simulink model "distributed_six"  (R2018a)
settings: Solver=VariableStepAuto  StartTime=0.0  StopTime=3000  FixedStep=0.0125  RelTol=1e-3  EnableMultiTasking=on
PreLoadFcn:
  | t_sampling = 0.1;
undefined symbols (not defined in the file or in its folder): DiscIntNeverNeededParam
settings Model: Creator=Kevin_ME813  LastModifiedBy=Kevin_ME813
settings SolverCC: ConcurrentTasks=on
settings DataIOCC: SaveFormat=Array
settings OptimizationCC: EnhancedBackFolding=on  PassReuseOutputArgsAs=Individual arguments  MaxStackSize=64  OptimizeBlockOrder=speed  DifferentSizesBufferReuse=on  OptimizationCustomize=off
settings DebuggingCC: ParameterTunabilityLossMsg=error
settings HardwareCC: ProdBitPerLong=64  ProdHWDeviceType=Intel->x86-64 (Linux 64)
settings SFSimCC: MATLABDynamicMemAlloc=off
settings RTWCC: SystemTargetFile=ert.tlc  HardwareBoard=Robot Operating System (ROS)  TLCOptions="-aInlineSetEventsForThisBaseRateFcn=TLC_FALSE -aSuppressMultiTaskScheduler=TLC_FALSE  -aRateBasedStepFcn=0"  TemplateMakefile=ert_default_tmf  GenerateReport=on  Toolchain=Catkin  IncludeHyperlinkInReport=on  LaunchReport=on  TargetLang=C++  GenerateTraceInfo=on  GenerateTraceReport=on  GenerateTraceReportSl=on  GenerateTraceReportSf=on  GenerateTraceReportEml=on
settings CodeAppCC: ForceParamTrailComments=on  IgnoreCustomStorageClasses=off  OperatorAnnotations=on  SimulinkDataObjDesc=on  SFDataObjDesc=on  InsertBlockDesc=on

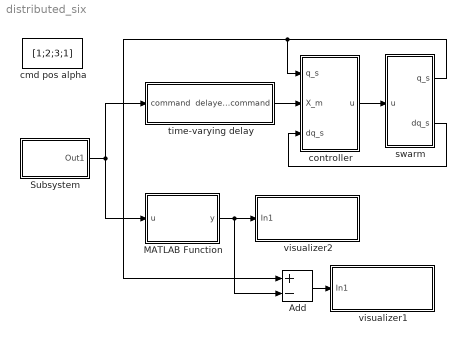
== system distributed_six ==
  Add : Sum  Inputs=+-
  MATLAB Function : MATLAB Function  TreatAsAtomicUnit=on
  Subsystem : Subsystem
  cmd pos alpha : Constant  Value=[1;2;3;1]  SampleTime=0.01
  controller : Subsystem
  swarm : Subsystem
  time-varying delay : Subsystem
  visualizer1 : Subsystem
  visualizer2 : Subsystem
  wires:
  swarm/1(q_s) -> Add/1, controller/1(q_s)
  swarm/2(dq_s) -> controller/3(dq_s)
  controller/1(u) -> swarm/1(u)
  time-varying delay/1(delayed command) -> controller/2(X_m)
  MATLAB Function/1(y) -> Add/2, visualizer2/1(In1)
  Add/1 -> visualizer1/1(In1)
  Subsystem/1(Out1) -> time-varying delay/1(command), MATLAB Function/1(u)

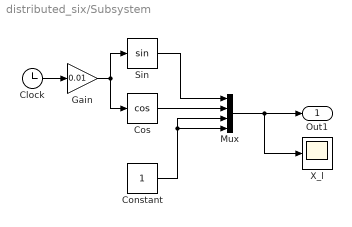
== system distributed_six/Subsystem ==
  Clock : Clock
  Constant : Constant  SampleTime=0.01
  Cos : Trigonometry  Operator=cos
  Gain : Gain  Gain=0.01
  Mux : Mux
  Sin : Trigonometry
  X_l : Scope
  Out1 : Outport
  wires:
  Mux/1 -> X_l/1, Out1/1
  Constant/1 -> Mux/3, Mux/4
  Cos/1 -> Mux/2
  Clock/1 -> Gain/1
  Sin/1 -> Mux/1
  Gain/1 -> Cos/1, Sin/1

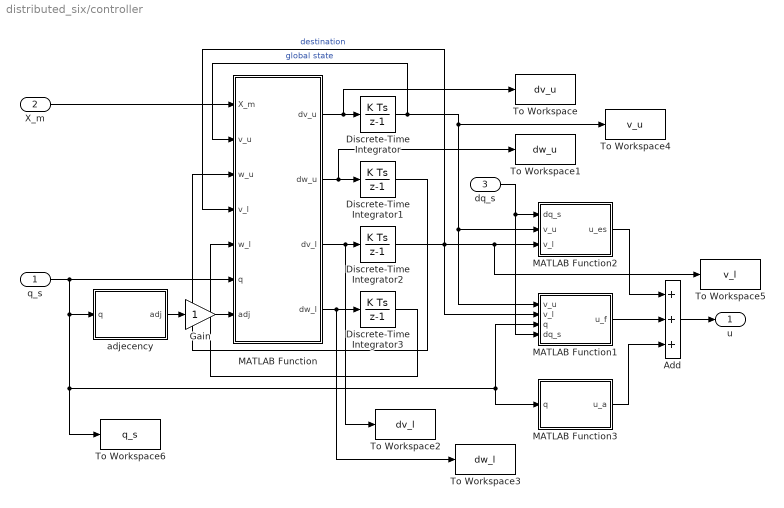
== system distributed_six/controller ==
  q_s : Inport
  X_m : Inport  Port=2
  dq_s : Inport  Port=3
  Add : Sum  Inputs=+++
  Discrete-Time Integrator{,1..3} (4 alike) : DiscreteIntegrator  SampleTime=-1  ICPrevOutput=DiscIntNeverNeededParam  ICPrevScaledInput=DiscIntNeverNeededParam
  Gain : Gain
  MATLAB Function : MATLAB Function  TreatAsAtomicUnit=on
  MATLAB Function1 : MATLAB Function  TreatAsAtomicUnit=on
  MATLAB Function2 : MATLAB Function  TreatAsAtomicUnit=on
  MATLAB Function3 : MATLAB Function  TreatAsAtomicUnit=on
  To Workspace : ToWorkspace  VariableName=dv_u  SampleTime=-1
  To Workspace1 : ToWorkspace  VariableName=dw_u  SampleTime=-1
  To Workspace2 : ToWorkspace  VariableName=dv_l  SampleTime=-1
  To Workspace3 : ToWorkspace  VariableName=dw_l  SampleTime=-1
  To Workspace4 : ToWorkspace  VariableName=v_u  SampleTime=-1
  To Workspace5 : ToWorkspace  VariableName=v_l  SampleTime=-1
  To Workspace6 : ToWorkspace  VariableName=q_s  SampleTime=-1
  adjecency : MATLAB Function  TreatAsAtomicUnit=on
  u : Outport
  wires:
  Discrete-Time Integrator1/1 -> MATLAB Function/3(w_u)
  q_s/1 -> To Workspace6/1, MATLAB Function3/1(q), MATLAB Function1/3(q), adjecency/1(q), MATLAB Function/6(q)
  Discrete-Time Integrator3/1 -> MATLAB Function/5(w_l)
  Discrete-Time Integrator2/1 -> To Workspace5/1, MATLAB Function2/3(v_l), MATLAB Function1/2(v_l), MATLAB Function/4(v_l)  "destination"
  MATLAB Function/3(dv_l) -> Discrete-Time Integrator2/1, To Workspace2/1
  MATLAB Function/4(dw_l) -> Discrete-Time Integrator3/1, To Workspace3/1
  Add/1 -> u/1
  MATLAB Function/2(dw_u) -> Discrete-Time Integrator1/1, To Workspace1/1
  Discrete-Time Integrator/1 -> To Workspace4/1, MATLAB Function1/1(v_u), MATLAB Function2/2(v_u), MATLAB Function/2(v_u)  "global state"
  MATLAB Function/1(dv_u) -> Discrete-Time Integrator/1, To Workspace/1
  MATLAB Function2/1(u_es) -> Add/1
  MATLAB Function3/1(u_a) -> Add/3
  dq_s/1 -> MATLAB Function1/4(dq_s), MATLAB Function2/1(dq_s)
  X_m/1 -> MATLAB Function/1(X_m)
  adjecency/1(adj) -> Gain/1
  Gain/1 -> MATLAB Function/7(adj)
  MATLAB Function1/1(u_f) -> Add/2

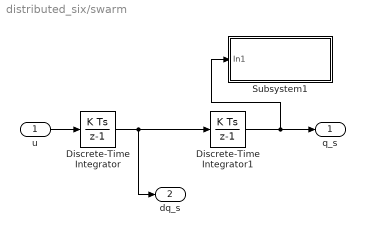
== system distributed_six/swarm ==
  u : Inport
  Discrete-Time Integrator : DiscreteIntegrator  InitialCondition=zeros(18,1)  SampleTime=-1  ICPrevOutput=DiscIntNeverNeededParam  ICPrevScaledInput=DiscIntNeverNeededParam
  Discrete-Time Integrator1 : DiscreteIntegrator  InitialCondition=[1 0 0 0.7 0.7 0 -0.7 0.7 0 -1 0 0 -0.7 -0.7 0 0.7 -0.7 0].'  SampleTime=-1  ICPrevOutput=DiscIntNeverNeededParam  ICPrevScaledInput=DiscIntNeverNeededParam
  Subsystem1 : Subsystem
  q_s : Outport
  dq_s : Outport  Port=2
  wires:
  u/1 -> Discrete-Time Integrator/1
  Discrete-Time Integrator/1 -> Discrete-Time Integrator1/1, dq_s/1
  Discrete-Time Integrator1/1 -> Subsystem1/1(In1), q_s/1

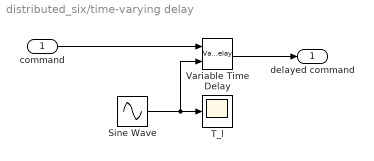
== system distributed_six/time-varying delay ==
  command : Inport
  Sine Wave : Sin  Amplitude=0.5  Bias=0.5  SampleTime=0
  T_l : Scope
  Variable Time Delay : VariableTransportDelay  MaximumDelay=5
  delayed command : Outport
  wires:
  Sine Wave/1 -> Variable Time Delay/2, T_l/1
  Variable Time Delay/1 -> delayed command/1
  command/1 -> Variable Time Delay/1

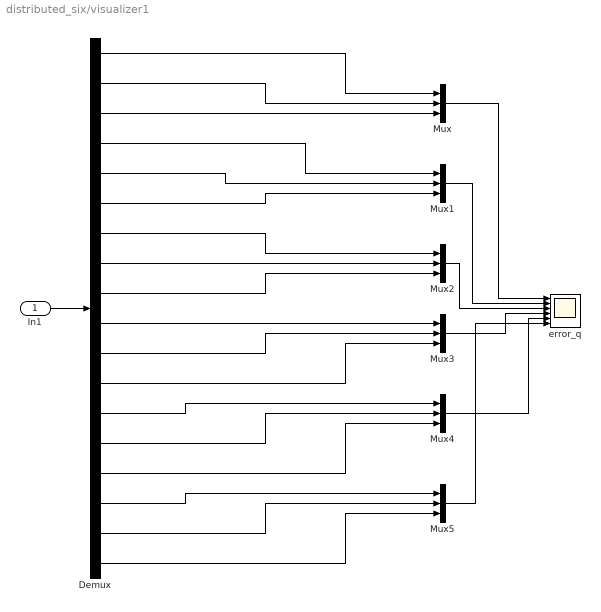
== system distributed_six/visualizer1 ==
  In1 : Inport
  Demux : Demux  Outputs=18
  Mux{,1..5} (6 alike) : Mux  Inputs=3
  error_q : Scope  NumInputPorts=6
  wires:
  Mux5/1 -> error_q/6
  Mux4/1 -> error_q/5
  Mux3/1 -> error_q/4
  Mux2/1 -> error_q/3
  Mux1/1 -> error_q/2
  Mux/1 -> error_q/1
  Demux/18 -> Mux5/3
  Demux/17 -> Mux5/2
  Demux/16 -> Mux5/1
  Demux/15 -> Mux4/3
  Demux/14 -> Mux4/2
  Demux/13 -> Mux4/1
  Demux/12 -> Mux3/3
  Demux/11 -> Mux3/2
  Demux/10 -> Mux3/1
  Demux/9 -> Mux2/3
  Demux/7 -> Mux2/1
  Demux/8 -> Mux2/2
  Demux/4 -> Mux1/1
  Demux/6 -> Mux1/3
  Demux/5 -> Mux1/2
  Demux/1 -> Mux/1
  Demux/2 -> Mux/2
  Demux/3 -> Mux/3
  In1/1 -> Demux/1

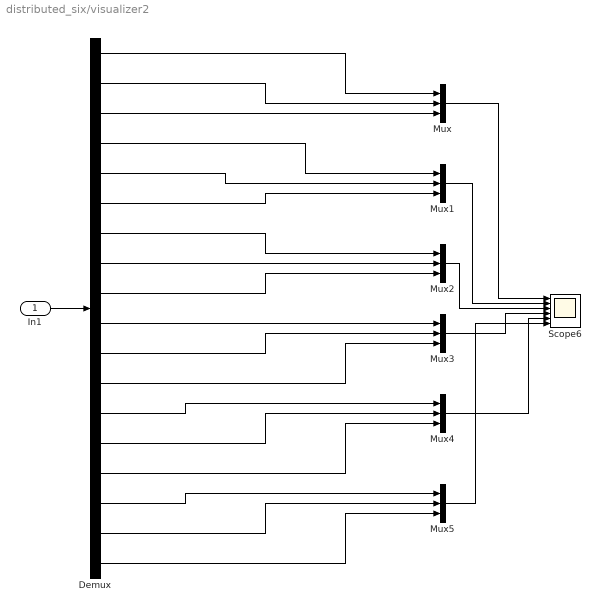
== system distributed_six/visualizer2 ==
  In1 : Inport
  Demux : Demux  Outputs=18
  Mux{,1..5} (6 alike) : Mux  Inputs=3
  Scope6 : Scope  NumInputPorts=6
  wires:
  In1/1 -> Demux/1
  Demux/3 -> Mux/3
  Demux/2 -> Mux/2
  Demux/1 -> Mux/1
  Demux/5 -> Mux1/2
  Demux/6 -> Mux1/3
  Demux/4 -> Mux1/1
  Demux/8 -> Mux2/2
  Demux/7 -> Mux2/1
  Demux/9 -> Mux2/3
  Demux/10 -> Mux3/1
  Demux/11 -> Mux3/2
  Demux/12 -> Mux3/3
  Demux/13 -> Mux4/1
  Demux/14 -> Mux4/2
  Demux/15 -> Mux4/3
  Demux/16 -> Mux5/1
  Demux/17 -> Mux5/2
  Demux/18 -> Mux5/3
  Mux/1 -> Scope6/1
  Mux1/1 -> Scope6/2
  Mux2/1 -> Scope6/3
  Mux3/1 -> Scope6/4
  Mux4/1 -> Scope6/5
  Mux5/1 -> Scope6/6

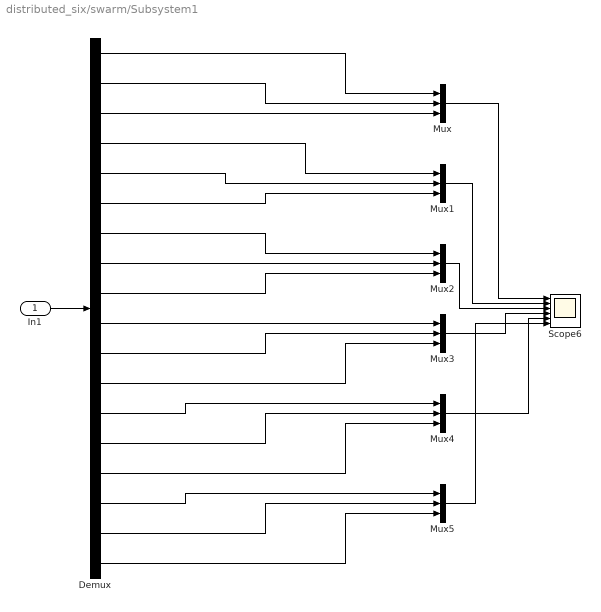
== system distributed_six/swarm/Subsystem1 ==
  In1 : Inport
  Demux : Demux  Outputs=18
  Mux{,1..5} (6 alike) : Mux  Inputs=3
  Scope6 : Scope  NumInputPorts=6
  wires:
  In1/1 -> Demux/1
  Demux/3 -> Mux/3
  Demux/2 -> Mux/2
  Demux/1 -> Mux/1
  Demux/5 -> Mux1/2
  Demux/6 -> Mux1/3
  Demux/4 -> Mux1/1
  Demux/8 -> Mux2/2
  Demux/7 -> Mux2/1
  Demux/9 -> Mux2/3
  Demux/10 -> Mux3/1
  Demux/11 -> Mux3/2
  Demux/12 -> Mux3/3
  Demux/13 -> Mux4/1
  Demux/14 -> Mux4/2
  Demux/15 -> Mux4/3
  Demux/16 -> Mux5/1
  Demux/17 -> Mux5/2
  Demux/18 -> Mux5/3
  Mux/1 -> Scope6/1
  Mux1/1 -> Scope6/2
  Mux2/1 -> Scope6/3
  Mux3/1 -> Scope6/4
  Mux4/1 -> Scope6/5
  Mux5/1 -> Scope6/6

== matlab function distributed_six/controller/adjecency ==
  data: q input; adj output
function adj = adjecency(q)
SlaveRobotNum = 6;
SlaveRobotDOF = 3;
DistanceLimit = 10;

reachable = zeros(SlaveRobotNum, SlaveRobotNum);
position = zeros(SlaveRobotNum, SlaveRobotDOF);

for num = 1 : SlaveRobotNum
    for axis = 1 : SlaveRobotDOF
        position(num, axis) = q( (num-1)*SlaveRobotDOF + axis);    
    end
end

for i = 1 : SlaveRobotNum
    for j = 1 : SlaveRobotNum
        
        if i == j
            reachable(i,j) = 0;
        elseif norm(position(i,:) - position(j,:)) <= DistanceLimit
            reachable(i,j) = 1;
        else
            reachable(i,j) = 0;
        end
    
    end
end

adj = reachable;

== matlab function distributed_six/controller/MATLAB Function ==
  data: X_m input; v_u input; dv_u output; dw_u output; w_u input; v_l input; w_l input; q input; adj input; dv_l output; dw_l output
function [dv_u,dw_u, dv_l, dw_l] = Estimator(X_m, v_u, w_u, v_l, w_l, q, adj)
SlaveRobotNum = 6;
SlaveRobotDOF = 3;
gamma = 1;
rho = 1;
k_p = 25;
k_i = 10;

dv_u = zeros(length(q),1);
dw_u = zeros(length(q),1);
dv_l = zeros(length(q)+SlaveRobotNum,1);
dw_l = zeros(length(q)+SlaveRobotNum,1);
delta = zeros(SlaveRobotNum,1);
delta(1) = 1;

for i = 1 : SlaveRobotNum   %robot number
    %index
    i1 = (i-1) * SlaveRobotDOF + 1;
    i1e = i1 + SlaveRobotDOF - 1;
    i3 = (i-1) * (SlaveRobotDOF+1) + 1;
    i3e = i3 + SlaveRobotDOF;
    
    dv_u(i1:i1e) = gamma*k_p*(q(i1:i1e) - v_u(i1:i1e));
%     dv_l(i3:i3e) = -delta(i)*k_p*(v_l(i3:i3e)-rho*X_m) + delta(i)*k_i*w_l(i3:i3e);
    dv_l(i3:i3e) = -delta(i)*k_p*(v_l(i3:i3e)-rho*X_m);
%     dw_l(i3:i3e) = -delta(i)*k_i*(v_l(i3:i3e)-rho*X_m);
    dw_l(i3:i3e) = -k_i*w_l(i3:i3e);
    
    
    for j = 1 : SlaveRobotNum   %sigma, others
        i2 = (j-1) * SlaveRobotDOF + 1;
        i2e = i2 + SlaveRobotDOF - 1;
        i4 = (j-1) * (SlaveRobotDOF+1) + 1;
        i4e = i4 + SlaveRobotDOF;
    
        if adj(i, j) ~= 0
            %3.7
            dv_u(i1:i1e) = dv_u(i1:i1e) ...
                - adj(i,j)*k_p*(v_u(i1:i1e)-v_u(i2:i2e)) ...
                + adj(i,j)*k_i*(w_u(i1:i1e)-w_u(i2:i2e));
            %3.8
            dw_u(i1:i1e) = dw_u(i1:i1e) - adj(i,j)*k_i*(v_u(i1:i1e)-v_u(i2:i2e));
            %3.9
            dv_l(i3:i3e) = dv_l(i3:i3e) ...
                - adj(i,j)*k_p*(v_l(i3:i3e)-v_l(i4:i4e)) ...
                + adj(i,j)*k_i*(w_l(i3:i3e)-w_l(i4:i4e));
            %3.10
            dw_l(i3:i3e) = dw_l(i3:i3e) - adj(i,j)*k_i*(v_l(i3:i3e)-v_l(i4:i4e));
            
        end
    end
end

== matlab function distributed_six/controller/MATLAB Function2 ==
  data: dq_s input; u_es output; v_u input; v_l input
function u_es = fcn(dq_s, v_u, v_l)
SlaveRobotNum = 6;
SlaveRobotDOF = 3;
b = ones(SlaveRobotNum, 1);
u_es = zeros(length(dq_s), 1);
Gamma = 1;
Lambda = 1;

for i = 1:SlaveRobotNum
%     index, 'e' for end
    i1 = (i-1) * SlaveRobotDOF + 1;
    i1e = i1 + SlaveRobotDOF - 1; 
    i2 = (i-1) * (SlaveRobotDOF+1) + 1;
    i2e = i2 + SlaveRobotDOF - 1;   %leading G terms
    
    u_es(i1:i1e) = -b(i)*dq_s(i1:i1e) ...
        - eye(SlaveRobotDOF)*Gamma*(v_u(i1:i1e)-v_l(i2:i2e)) ...   %eye to be modified
        - Lambda * eye(SlaveRobotDOF) * dq_s(i1:i1e);
end

== matlab function distributed_six/controller/MATLAB Function1 ==
  data: v_u input; u_f output; v_l input; q input; dq_s input
function u_f = fcn(v_u, v_l, q, dq_s)
SlaveRobotNum = 6;
SlaveRobotDOF = 3;

q_d = zeros(length(q),1);
d_f = zeros(length(q),1);
d_f(1) = 1;
u_f = zeros(length(q),1);
k_f = 1;
k_fd = 0;

for i = 1 : SlaveRobotNum   %robot number
    %index
    i1 = (i-1) * SlaveRobotDOF + 1;
    i1e = i1 + SlaveRobotDOF - 1;
    i3 = (i-1) * (SlaveRobotDOF+1) + 1;
    i3e = i3 + SlaveRobotDOF;
          
    
    q_d(i1:i1e) = v_l(i3e)*d_f(i1:i1e) + v_u(i1:i1e);
    u_f(i1:i1e) = -k_f*( q(i1:i1e)-q_d(i1:i1e) )- k_fd*dq_s(i1:i1e);
    
    if i ~= SlaveRobotNum
        d_f(i1+SlaveRobotDOF:i1e+SlaveRobotDOF) ...
            = rotz(360/SlaveRobotNum)*d_f(i1:i1e);
    end
end

== matlab function distributed_six/controller/MATLAB Function3 ==
  data: q input; u_a output
function u_a = fcn(q)

u_a = 0;

== matlab function distributed_six/MATLAB Function ==
  data: u input; y output
function y = fcn(u)

y1 = u(1:3) + u(4)*[1;0;0];
y2 = u(1:3) + u(4)*[0.5;0.866;0];
y3 = u(1:3) + u(4)*[-0.5;0.866;0];
y4 = u(1:3) + u(4)*[-1;0;0];
y5 = u(1:3) + u(4)*[-0.5;-0.866;0];
y6 = u(1:3) + u(4)*[0.5;-0.866;0];

y = [y1;y2;y3;y4;y5;y6];
